simulink model "PV_Array_MPPT"  (R2021a)
settings: Solver=FixedStepAuto  StartTime=0.0  StopTime=10.0  FixedStep=5e-6  RelTol=1e-3
libraries: spsSeriesRLCBranchLib x5, spsCurrentMeasurementLib x1, spsDiodeLib x1, spsIGBTDiodeLib x1, spsPVArrayLib x1, spsPWMGeneratorDCDCLib x1, spsVoltageMeasurementLib x1, spspowerguiLib x1
settings Model: Creator=Anass Soulimani  LastModifiedBy=Anass Soulimani

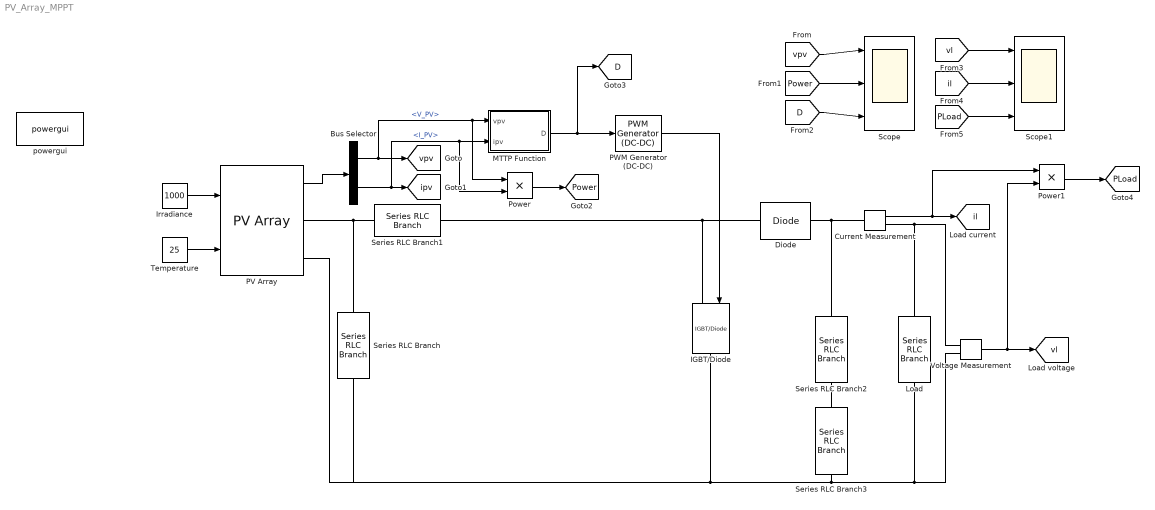
== system PV_Array_MPPT ==
  Bus Selector : BusSelector  OutputSignals=V_PV,I_PV
  Current Measurement : spsCurrentMeasurementLib/Current Measurement  PhasorSimulation=off  OutputType=Complex  PSBequivalent=0
  Diode : spsDiodeLib/Diode  Ron=0.001  Lon=0  Vf=0.8  IC=0  UseSnubber=0  Rs=500  Cs=250e-9  Measurements=off
  IGBT/Diode : spsIGBTDiodeLib/IGBT//Diode  Ron=1e-3  Rs=1e5  Cs=inf  Measurements=off
  Irradiance : Constant  Value=1000
  Load : spsSeriesRLCBranchLib/Series RLC Branch  LConnTagsString=__new0  RConnTagsString=__new0  BranchType=R  Resistance=10  Inductance=5e-3  SetiL0=off  InitialCurrent=0  Capacitance=12000e-6  Setx0=off  InitialVoltage=0  Measurements=None
  MTTP Function : MATLAB Function  TreatAsAtomicUnit=on
  PV Array : spsPVArrayLib/PV Array  Npar=64  Nser=5  PlotType=array @ 1000 W/m2 & specified temperatures  S_vec="[ 1000  500  100 ]"  Temp_C_vec="[ 45 25  ]"  ModuleName=SunPower SPR-315E-WHT-D  PlotWhenSelected=off  Pm=315.072  Ncell=96  Voc=64.6  Isc=6.14  Vm=54.7  Im=5.76  beta_Voc_pc=-0.2727  alpha_Isc_pc=0.061743  beta_Voc=-0.17616  alpha_Isc=0.003791  IL=6.1461  I0=6.5067e-12  nI=0.95071  Rsh=430.0666  Rs=0.43041  RobustModel=off  RobustCellTemperature=313.3991  BAL=on  Tc=1e-6  Tfilter=5e-5
  PWM Generator (DC-DC) : spsPWMGeneratorDCDCLib/PWM Generator (DC-DC)  Fsw=5000  Ts=5e-6
  Power : Product
  Power1 : Product
  Scope : Scope  NumInputPorts=3
  Scope1 : Scope  NumInputPorts=3
  Series RLC Branch : spsSeriesRLCBranchLib/Series RLC Branch  LConnTagsString=__new0  RConnTagsString=__new0  BranchType=C  Resistance=100  Inductance=1e-3  SetiL0=off  InitialCurrent=0  Capacitance=100e-6  Setx0=off  InitialVoltage=0  Measurements=None
  Series RLC Branch1 : spsSeriesRLCBranchLib/Series RLC Branch  LConnTagsString=__new0  RConnTagsString=__new0  BranchType=L  Resistance=100  Inductance=5e-3  SetiL0=off  InitialCurrent=0  Capacitance=100e-6  Setx0=off  InitialVoltage=0  Measurements=None
  Series RLC Branch2 : spsSeriesRLCBranchLib/Series RLC Branch  LConnTagsString=__new0  RConnTagsString=__new0  BranchType=C  Resistance=100  Inductance=5e-3  SetiL0=off  InitialCurrent=0  Capacitance=12000e-6  Setx0=off  InitialVoltage=0  Measurements=None
  Series RLC Branch3 : spsSeriesRLCBranchLib/Series RLC Branch  LConnTagsString=__new0  RConnTagsString=__new0  BranchType=C  Resistance=100  Inductance=5e-3  SetiL0=off  InitialCurrent=0  Capacitance=12000e-6  Setx0=off  InitialVoltage=0  Measurements=None
  Temperature : Constant  Value=25
  Voltage Measurement : spsVoltageMeasurementLib/Voltage Measurement  PhasorSimulation=off  OutputType=Complex  PSBequivalent=0
  powergui : spspowerguiLib/powergui  Priority=1  SimulationMode=Discrete  SampleTime=5e-6  frequency=60  Iterations=50  frequencyindice=0  Pbase=100e6  ErrMax=1e-4  UnitsV=kV  UnitsW=MW  buscounter=0  FunctionMessages=off  echomessages=off  EnableUseOfTLC=off  CurrentSourceSwitches=off  DisableSnubberDevices=off  DisableRonSwitches=off  DisableVfSwitches=off  DisplayEquations=off  AutomaticDiscreteSolvers=off  SolverType=Tustin/Backward Euler (TBE)  Interpol=off  ExternalGateDelay=off  methode=off  Ts=100  x0status=blocks  SPID=on  SwTol=0  HookPort=off  NonlinearTolerance=1e-4  nMaxIteration=100  ContinueOnMaxIteration=off  RestoreLinks=warning  ResistiveCurrentMeasurement=off  Frange=[0:2:500]  Ylog=off  Xlog=on  ShowGrid=off  save=off  variable=ZData  structure=0  ZoomFFT=off  StartTime=0.0  cycles=1  DisplayStyle=1  fundamental=60  FreqAxis=off  MaxFrequency=1000  frequencyindicesteady=1  RmsSteady=1  display=off
  tag scope: D=global, PLoad=global, Power=global, il=global, ipv=global, vl=global, vpv=global
  wires:
  PV Array/1 -> Bus Selector/1
  Bus Selector/1 -> Power/1, MTTP Function/1(vpv), [vpv]  "<V_PV>"
  Bus Selector/2 -> Power/2, MTTP Function/2(ipv), [ipv]  "<I_PV>"
  Voltage Measurement/1 -> [vl], Power1/2
  Current Measurement/1 -> Power1/1, [il]
  Irradiance/1 -> PV Array/1
  Temperature/1 -> PV Array/2
  MTTP Function/1(D) -> [D], PWM Generator (DC-DC)/1
  PWM Generator (DC-DC)/1 -> IGBT/Diode/1
  Power/1 -> [Power]
  Power1/1 -> [PLoad]
  [vpv] -> Scope/1
  [Power] -> Scope/2
  [D] -> Scope/3
  [vl] -> Scope1/1
  [il] -> Scope1/2
  [PLoad] -> Scope1/3
  connections:
  PV Array/RConn1 -- Series RLC Branch/LConn1 -- Series RLC Branch1/RConn1
  Series RLC Branch1/LConn1 -- IGBT/Diode/LConn1 -- Diode/LConn1
  Series RLC Branch3/RConn1 -- Series RLC Branch2/LConn1
  Load/LConn1 -- Voltage Measurement/LConn2 -- Series RLC Branch3/LConn1 -- Series RLC Branch/RConn1 -- PV Array/RConn2 -- IGBT/Diode/RConn1
  Voltage Measurement/LConn1 -- Load/RConn1 -- Current Measurement/RConn1
  Series RLC Branch2/RConn1 -- Current Measurement/LConn1 -- Diode/RConn1

== matlab function PV_Array_MPPT/MTTP Function ==
  data: vpv input; D output; ipv input
function D = fcn(vpv,ipv)
Dinit = 0.4;
Dmax = 0.9;
Dmin = 0.1;
deltaD = 20e-6;

persistent Vold Pold Dold;

dataType = "double";

if isempty(Vold)
    Vold = 0;
    Pold = 0;
    Dold = Dinit;
end

P = vpv * ipv;
dV = vpv - Vold;
dP = P - Pold;

if dP ~= 0
    if dP < 0
        if dV < 0
            D = Dold - deltaD;
        else
            D = Dold + deltaD;
        end
    else
        if dV < 0
            D = Dold + deltaD;
        else
            D = Dold - deltaD;
        end
    end
else
    D = Dold;
end
if D >= Dmax | D <= Dmin
    D = Dold;
end

Dold = D;
Vold = vpv;
Pold = P;
